simulink model "Chem_E_Car_System_LDR_PT"  (R2026a)
settings: Solver=VariableStepAuto  AbsTol=1e-3
libraries: fl_lib x32, ElectroChem_lib x10, nesl_utility x9, ee_lib x7, batteryecm_lib x1, batt_lib x1, sdl_lib x1
settings Model: Creator=eyede  LastModifiedBy=davin
settings DebuggingCC: SymbolicDimsDataTypeCodeGenerationDiagnostic=none
settings SimscapeCC: SimscapeNominalValues="[{\"value\":\"1\",\"unit\":\"A\"},{\"value\":\"1\",\"unit\":\"bar\"},{\"value\":\"1\",\"unit\":\"cm^2\"},{\"value\":\"1\",\"unit\":\"cm^3/s\"},{\"value\":\"1\",\"unit\":\"kJ/kg\"},{\"value\":\"1\",\"unit\":\"kW\"},{\"value\":\"1\",\"unit\":\"l\"},{\"value\":\"1\",\"unit\":\"N\"},{\"value\":\"1\",\"unit\":\"N*m\"},{\"value\":\"1\",\"unit\":\"V\"}]"  SimscapeLogSimulationStatistics=on

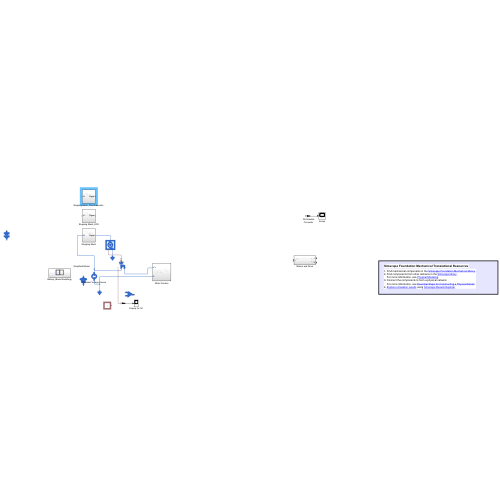
[thumbnail: Simulink's stored preview of the top-level diagram]
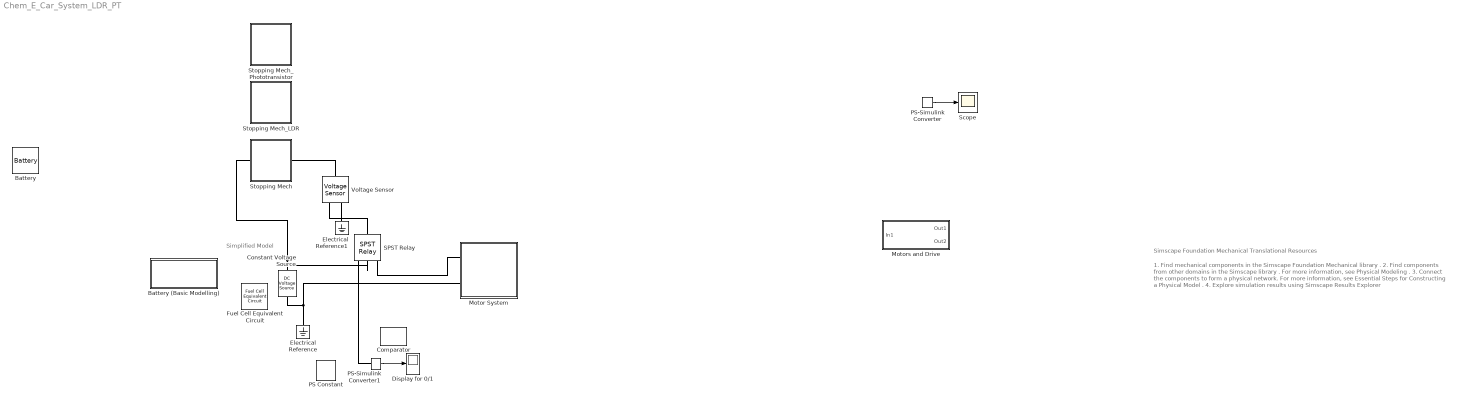
== system Chem_E_Car_System_LDR_PT ==
  note: Simplified Model
  note: 1. Find mechanical components in the Simscape Foundation Mechanical library .
      | 2. Find components from other domains in the Simscape library .
      | For more information, see Physical Modeling .
      | 3. Connect the components to form a physical network.
      | For more information, see Essential Steps for Constructing a Physical Model .
      | 4. Explore simulation results using Simscape Results Explorer
  note: Simscape Foundation Mechanical Translational Resources
  Battery : batteryecm_lib/Battery  Vnom=12 V  prm_dir=simscape.enum.battery.prm_dir.disabled  R1_dis=2 Ohm  R1_ch=2 Ohm  R1=2 Ohm  prm_AH=simscape.enum.battery.prm_AH.infinite  AH=50 A*hr  V1=11.5 V  AH1=25 A*hr  prm_R2=simscape.enum.battery.prm_R2.disabled  R2=2000 Ohm  Tmeas=298.15 K  charge_measurement_port=simscape.enum.battery.enable.no  prm_dyn=simscape.enum.battery.prm_dyn.off  Rp1=0.005 Ohm  tau1=30 s  Rp2=0.005 Ohm  tau2=30 s  Rp3=0.005 Ohm  tau3=30 s  Rp4=0.005 Ohm  tau4=30 s  Rp5=0.005 Ohm  tau5=30 s  prm_fade=simscape.enum.battery.prm_fade.disabled  N_fade=100  AH_fade=45 A*hr  R1_fade=2.02 Ohm  R1_ch_fade=2.02 Ohm  V1_fade=10.35 V  prm_age=simscape.enum.battery.prm_age.disabled  prm_age_OCV=simscape.enum.battery.prm_age_OCV.OCV  OCV_age=0.9  SOC_age=60  Tmeas_age=298.15 K  delta_time_age_vec=[0] d  temperature_age_vec=[273] K  OCV_scaling_age=2.2134e6  OCV_offset_age=1.632e6  temp_exp_age=0.515833569 V  t_exp_age=0.75  Vnom_T2=12 V  R1_T2=2.2 Ohm  R1_T2_dis=2.2 Ohm  R1_T2_ch=2.2 Ohm  V1_T2=11.4 V  R2_T2=2200 Ohm  Rp1_T2=0.005 Ohm  tau1_T2=30 s  Rp2_T2=0.005 Ohm  tau2_T2=30 s  Rp3_T2=0.005 Ohm  tau3_T2=30 s  Rp4_T2=0.005 Ohm  tau4_T2=30 s  Rp5_T2=0.005 Ohm  tau5_T2=30 s  Tmeas2=273.15 K  thermal_port=simscape.enum.thermaleffects.omit  thermal_mass=30000 J/K  i_specify=off  i_priority=None  i=0 A  i_nominal_specify=off  i_nominal_value=1  i_nominal_unit=A  v_specify=off  v_priority=None  v=0 V  v_nominal_specify=off  v_nominal_value=1  v_nominal_unit=V  charge_specify=off  charge_priority=High  charge=50 A*hr  charge_nominal_specify=off  charge_nominal_value=1  charge_nominal_unit=A*hr  num_cycles_specify=off  num_cycles_priority=High  num_cycles=0  num_cycles_nominal_specify=off  num_cycles_nominal_value=1  num_cycles_nominal_unit=1  temperature_specify=off  temperature_priority=High  temperature=298.15 K  temperature_nominal_specify=off  temperature_nominal_value=1  temperature_nominal_unit=K
  Battery (Basic Modelling) : Subsystem
  Comparator : ee_lib/Integrated Circuits/Comparator  V_OS=5 mV  C_IN=0 pF  V_OL=0 V  V_OH=5 V  R_OUT=50 Ohm  Delay=0 s
  Constant Voltage Source : ee_lib/Additional Components/SPICE Sources/DC Voltage Source  DC=6 V
  Display for 0/1 : Display
  Electrical Reference : fl_lib/Electrical/Electrical Elements/Electrical Reference
  Electrical Reference1 : fl_lib/Electrical/Electrical Elements/Electrical Reference
  Fuel Cell Equivalent Circuit : batt_lib/Cells/Fuel Cell Equivalent Circuit  Area=14.8 cm^2  NominalPotential=6 V  VoltageRange=[0, inf] V  TafelSlope=0.0136 V  NominalExchangeCurrent=0.04777 A  EquivalentResistanceRC=5e-3 Ohm  TimeConstantRC=100 s  Thickness=0.127 mm  Density=1.9 g/cm^3  MolarMass=1400 g/mol  NumSlices=3  MoistureSpec=simscape.battery.enum.cells.MoistureSpec.lambda  LambdaInterface=simscape.battery.enum.cells.BlockInterface.parameters  RHAnodeParameter=1  RHCathodeParameter=1  LambdaAnodeParameter=1  LambdaCathodeParameter=1  InitialRH=1  InitialLambda=1  DiffusionInterface=simscape.battery.enum.cells.BlockCoefficientInterface.parameters  DiffusionCoefficient=1.5e-10 m^2/s  DiffusionTableData=[1e-10, 1.5e-10] m^2/s  DiffusionBreakpoints=[0, 400] K  DragInterface=simscape.battery.enum.cells.BlockCoefficientInterface.parameters  DragCoefficient=2.5  DragTableData=[1, 2.5, 2.5]  DragBreakpoints=[1, 14, 20]  DragScaleFactor=1  TemperatureInterface=simscape.battery.enum.cells.BlockInterface.parameters  CellTemperatureParameter=303.15 K  fuelCellVoltage_specify=off  fuelCellVoltage_priority=None  fuelCellVoltage=0 V  fuelCellVoltage_nominal_specify=off  fuelCellVoltage_nominal_value=1  fuelCellVoltage_nominal_unit=V  fuelCellCurrent_specify=off  fuelCellCurrent_priority=None  fuelCellCurrent=0 A  fuelCellCurrent_nominal_specify=off  fuelCellCurrent_nominal_value=1  fuelCellCurrent_nominal_unit=A
  Motor System : Subsystem
  Motors and Drive : Subsystem
  PS Constant : fl_lib/Physical Signals/Sources/PS Constant  constant=1
  PS-Simulink Converter : nesl_utility/PS-Simulink Converter  PhysicalDomain=network_engine_domain  SubClassName=ps_output  LeftPortType=input  RightPortType=output  PseudoPeriodic=off  Frequencies=[]  VectorFormat=inherit  Unit=inherit  AffineConversion=off
  PS-Simulink Converter1 : nesl_utility/PS-Simulink Converter  PhysicalDomain=network_engine_domain  SubClassName=ps_output  LeftPortType=input  RightPortType=output  PseudoPeriodic=off  Frequencies=[]  VectorFormat=inherit  Unit=inherit  AffineConversion=off
  SPST Relay : ee_lib/Switches & Breakers/Relays/SPST Relay  block_choices=ee.enum.controlport.ps  R_closed=0 Ohm  G_open=1e-8 1/Ohm  Threshold=1  exposemeasurement=ee.enum.exposemeasurement.visible  V_rated=5 V  V_energize=75  V_deenergize=25  l_winding=0.08 H  r_winding=12.5 Ohm  g_winding=1e-9 1/Ohm  T_brk_C_S=0 s  T_mak_C_S=0 s  fault_types=ee.enum.relays.faultTypes.winding
  Scope : Scope
  Stopping Mech : Subsystem
  Stopping Mech_LDR : Subsystem
  "Stopping Mech_Phototransistor " : Subsystem
  Voltage Sensor : fl_lib/Electrical/Electrical Sensors/Voltage Sensor
  wires:
  PS-Simulink Converter/1 -> Scope/1
  PS-Simulink Converter1/1 -> Display for 0/1/1
  connections:
  Electrical Reference/LConn1 -- Motor System/LConn2 -- Constant Voltage Source/RConn1
  Voltage Sensor/LConn1 -- Stopping Mech/RConn1
  SPST Relay/RConn1 -- Motor System/LConn1
  SPST Relay/RConn2 -- Stopping Mech/LConn1 -- Constant Voltage Source/LConn1
  Voltage Sensor/RConn1 -- SPST Relay/LConn1
  Electrical Reference1/LConn1 -- Voltage Sensor/RConn2
  PS-Simulink Converter1/LConn1 -- SPST Relay/RConn3

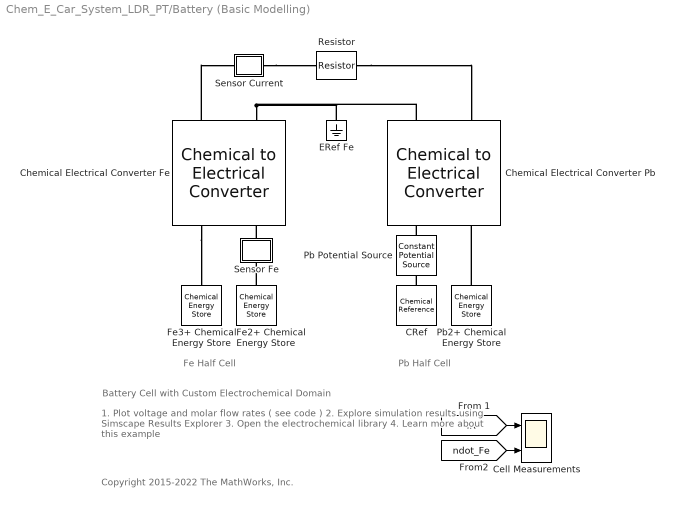
== system Chem_E_Car_System_LDR_PT/Battery (Basic Modelling) ==
  note: 1. Plot voltage and molar flow rates ( see code )
      | 2. Explore simulation results using Simscape Results Explorer
      | 3. Open the electrochemical library
      | 4. Learn more about this example
  note: Battery Cell with Custom Electrochemical Domain
  note: Copyright 2015-2022 The MathWorks, Inc.
  note: Pb Half Cell
  note: Fe Half Cell
  CRef : ElectroChem_lib/Electrochemical Elements/Chemical Reference
  Cell Measurements : Scope  NumInputPorts=2
      settings: Title=Battery Current (A)  ActiveDisplayYMinimum=-0.0017010196663266859  ActiveDisplayYMaximum=100  DataLoggingSaveFormat=Array
  Chemical Electrical Converter Fe : ElectroChem_lib/Electrochemical Elements/Chemical to Electrical Converter  z=1  i_specify=off  i_priority=High  i=0 A  i_nominal_specify=off  i_nominal_value=1  i_nominal_unit=A  ndot_specify=off  ndot_priority=High  ndot=0 mol/s  ndot_nominal_specify=off  ndot_nominal_value=1  ndot_nominal_unit=mol/s
  Chemical Electrical Converter Pb : ElectroChem_lib/Electrochemical Elements/Chemical to Electrical Converter  z=2  i_specify=off  i_priority=High  i=0 A  i_nominal_specify=off  i_nominal_value=1  i_nominal_unit=A  ndot_specify=off  ndot_priority=High  ndot=0 mol/s  ndot_nominal_specify=off  ndot_nominal_value=1  ndot_nominal_unit=mol/s
  ERef Fe : fl_lib/Electrical/Electrical Elements/Electrical Reference
  Fe2+ Chemical Energy Store : ElectroChem_lib/Electrochemical Elements/Chemical Energy Store  mu0=-78.87e3 J/mol  m_solvent=1 kg  T=298 K  ndot_specify=off  ndot_priority=High  ndot=0 mol/s  ndot_nominal_specify=off  ndot_nominal_value=1  ndot_nominal_unit=mol/s  n_specify=on  n_priority=High  n=0.01 mol  n_nominal_specify=off  n_nominal_value=1  n_nominal_unit=mol
  Fe3+ Chemical Energy Store : ElectroChem_lib/Electrochemical Elements/Chemical Energy Store  mu0=-4.60e3 J/mol  m_solvent=1 kg  T=298 K  ndot_specify=off  ndot_priority=High  ndot=0 mol/s  ndot_nominal_specify=off  ndot_nominal_value=1  ndot_nominal_unit=mol/s  n_specify=on  n_priority=High  n=0.05 mol  n_nominal_specify=off  n_nominal_value=1  n_nominal_unit=mol
  Pb Potential Source : ElectroChem_lib/Electrochemical Sources/Constant Potential Source  mu0=0 J/mol
  Pb2+ Chemical Energy Store : ElectroChem_lib/Electrochemical Elements/Chemical Energy Store  mu0=-24.39e3 J/mol  m_solvent=1 kg  T=298 K  ndot_specify=off  ndot_priority=High  ndot=0 mol/s  ndot_nominal_specify=off  ndot_nominal_value=1  ndot_nominal_unit=mol/s  n_specify=on  n_priority=High  n=0.1 mol  n_nominal_specify=off  n_nominal_value=1  n_nominal_unit=mol
  Resistor : fl_lib/Electrical/Electrical Elements/Resistor  R=0.012 Ohm  i_specify=off  i_priority=High  i=0 A  i_nominal_specify=off  i_nominal_value=1  i_nominal_unit=A  v_specify=off  v_priority=High  v=0 V  v_nominal_specify=off  v_nominal_value=1  v_nominal_unit=V
  Sensor Current : Subsystem
      mask Display: disp('iR')
  Sensor Fe : Subsystem
      mask Display: disp('ndot')
  wires:
  [ndot_Fe] -> Cell Measurements/2
  [iR] -> Cell Measurements/1
  connections:
  Chemical Electrical Converter Fe/LConn2 -- ERef Fe/LConn1 -- Chemical Electrical Converter Pb/LConn2
  Pb Potential Source/LConn1 -- Chemical Electrical Converter Pb/RConn2
  Resistor/RConn1 -- Chemical Electrical Converter Pb/LConn1
  Chemical Electrical Converter Fe/RConn1 -- Fe3+ Chemical Energy Store/LConn1
  CRef/LConn1 -- Pb Potential Source/RConn1
  Fe2+ Chemical Energy Store/LConn1 -- Sensor Fe/RConn1
  Chemical Electrical Converter Fe/LConn1 -- Sensor Current/LConn1
  Sensor Fe/LConn1 -- Chemical Electrical Converter Fe/RConn2
  Sensor Current/RConn1 -- Resistor/LConn1
  Pb2+ Chemical Energy Store/LConn1 -- Chemical Electrical Converter Pb/RConn1

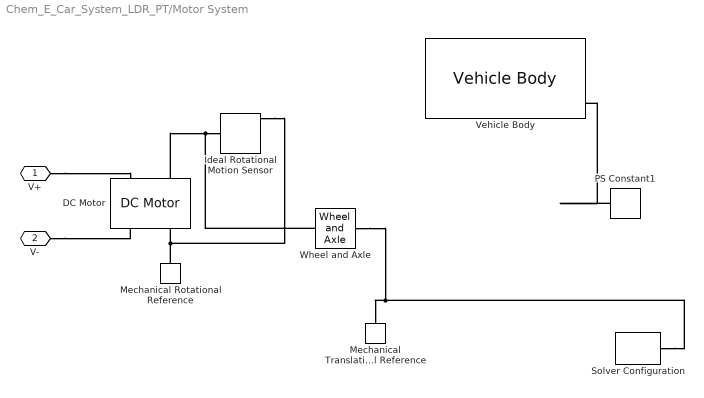
== system Chem_E_Car_System_LDR_PT/Motor System ==
  DC Motor : ee_lib/Electromechanical/Brushed Motors/DC Motor  field_option=ee.enum.field_option.pm  Rf=100 Ohm  Lf=1 H  Laf=0.15 H  If0=0 A  parameterization=ee.enum.dcparam_option.circuit_param  Ra=3.9 Ohm  La=12e-6 H  emf_or_torque=ee.enum.emf_or_torque.kv  Kv=0.072e-3 V/rpm  Ki=6.876e-4 N*m/A  T_stall=0.24e-3 N*m  w_max=19100 rpm  w_rated=15000 rpm  P_rated=0.08 W  V_rated=1.5 V  lam_param=ee.enum.lam_param.damping  i_noload=0 A  V_i_noload=1.5 V  J=0.01 cm^2*g  lam=0 N*m*s/rad  speed0=0 rpm  alpha=3.93e-3 1/K  Tmeas=25 degC  thermal_mass=100 J/K  initial_temperature=25 degC
  Ideal Rotational Motion Sensor : fl_lib/Mechanical/Mechanical Sensors/Ideal Rotational Motion Sensor  reference=foundation.enum.MeasurementReference.difference  acceleration_port=false  velocity_port=true  position_port=true  wrap_angle=false  offset=0 rad
  Mechanical Rotational Reference : fl_lib/Mechanical/Rotational Elements/Mechanical Rotational Reference
  Mechanical Translational Reference : fl_lib/Mechanical/Translational Elements/Mechanical Translational Reference
  PS Constant1 : fl_lib/Physical Signals/Sources/PS Constant  constant=0
  Solver Configuration : nesl_utility/Solver Configuration  PhysicalDomain=network_engine_domain  SubClassName=solver  LeftPortType=input  RightPortType=generic  Tones=[]  Harmonics=[]  SimulateNoise=off  Profile=off  UseLocalSampling=off  EnableSwitchedLinearOptims=on  FrequencyDomain=off  UseCCode=off  RelTol=0.001  AbsTol=1e-06  MinStep=1e-09  ToWorkspace=off  RevertToSquareIcSolve=off  NumHomotopyIterations=100  PhasorMode=off  PhasorModeNumHarmonics=1  ConsistencySolver=NEWTON_XTOL_AFTER_FTOL  CanonicalOrdering=UNORDERED  OptimizeIntermediates=UNOPTIMIZED  IndexReductionMethod=DerivativeReplacement  DoDC=off  ResidualTolerance=1e-09  ConsistencyTolSource=GLOBAL  ConsistencyAbsTol=0.001  ConsistencyRelTol=0.001  ConsistencyTolFactor=0.001  UseLocalSolver=off  LocalSolverChoice=NE_BACKWARD_EULER_ADVANCER  ResolveIndetEquations=on  FunctionEvalNumThread=1  LocalSolverSampleTime=0.001  DoFixedCost=off  MaxNonlinIter=3  MaxModeIter=2  ComputeImpulses=off  ImpulseIterations=2  LinearAlgebra=auto  LinearAlgebraNumThread=0  EquationFormulation=NE_TIME_EF  DelaysMemoryBudget=1024  AutomaticFiltering=on  FilteringTimeConstant=0.001  PartitionStorageMethod=AS_NEEDED  PartitionMemoryBudget=1024  PartitionMethod=ROBUST  MultibodyUseLocalSolver=off  MultibodyLocalSolverChoice=ODE1  MultibodyLocalSolverSampleTime=0.001
  Vehicle Body : sdl_lib/Tires & Vehicles/Vehicle Body  mass=1200 kg  n_w=2  x_f=1.4 m  x_r=1.6 m  y_c=0.5 m  mass_var=false  g=9.81 m/s^2  liftoff_warning=false  area=3 m^2  Cd_var=false  Cd=0.4  rho=1.18 kg/m^3  model_pitch=false  inertia=4000 kg*m^2  suspension_model=sdl.enum.linearTLU.linear  k_f=1e4 N/m  b_f=1e4 N*s/m  k_r=1e4 N/m  b_r=1e4 N*s/m  k_f_TLU=[-2000, -1000, 0, 1000, 2000] N  x_f_TLU=[-.4, -.2, 0, .2, .4] m  b_f_TLU=[-200, -100, 0, 100, 200] N  v_f_TLU=[-4, -2, 0, 2, 4] m/s  k_r_TLU=[-2000, -1000, 0, 1000, 2000] N  x_r_TLU=[-.4, -.2, 0, .2, .4] m  b_r_TLU=[-200, -100, 0, 100, 200] N  v_r_TLU=[-4, -2, 0, 2, 4] m/s  interp_method=simscape.enum.interpolation.linear  extrap_method=simscape.enum.extrapolation.linear  model_hardstop=false  upper_bound_f=.25 m  lower_bound_f=-.25 m  stop_k_f=1e6 N/m  stop_b_f=150 N*s/m  upper_bound_r=.25 m  lower_bound_r=-.25 m  stop_k_r=1e6 N/m  stop_b_r=150 N*s/m  initial_pitch=0 rad  initial_pitch_rate=0 rad/s  v_specify=off  v_priority=High  v=0 m/s  v_nominal_specify=off  v_nominal_value=1  v_nominal_unit=m/s
  Wheel and Axle : fl_lib/Mechanical/Mechanisms/Wheel and Axle  R=0.05 m  or=foundation.enum.DriveOrientation.Positive  t_specify=off  t_priority=None  t=0 N*m  t_nominal_specify=off  t_nominal_value=1  t_nominal_unit=N*m  f_specify=off  f_priority=None  f=0 N  f_nominal_specify=off  f_nominal_value=1  f_nominal_unit=N
  V+ : PMIOPort  Side=Left
  V- : PMIOPort  Port=2  Side=Left
  connections:
  DC Motor/RConn2 -- Mechanical Rotational Reference/LConn1 -- Ideal Rotational Motion Sensor/RConn1
  Ideal Rotational Motion Sensor/LConn1 -- DC Motor/LConn2 -- Wheel and Axle/LConn1
  Solver Configuration/RConn1 -- Wheel and Axle/RConn1 -- Mechanical Translational Reference/LConn1
  PS Constant1/RConn1 -- Vehicle Body/RConn3
  V+/RConn1 -- DC Motor/LConn1
  V-/RConn1 -- DC Motor/RConn1

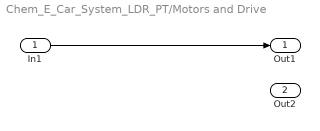
== system Chem_E_Car_System_LDR_PT/Motors and Drive ==
  In1 : Inport
  Out1 : Outport
  Out2 : Outport  Port=2
  wires:
  In1/1 -> Out1/1

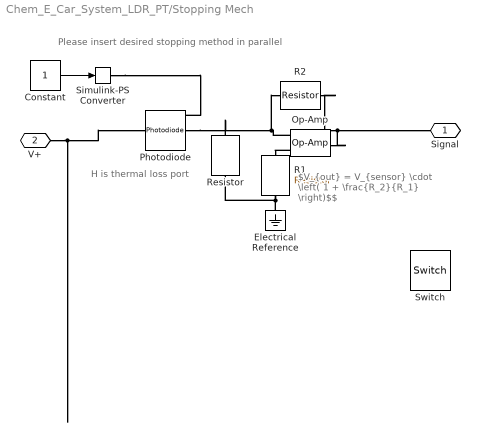
== system Chem_E_Car_System_LDR_PT/Stopping Mech ==
  note: $V_{out} = V_{sensor} \cdot \left( 1 + \frac{R_2}{R_1} \right)$$
  note: H is thermal loss port
  note: Please insert desired stopping method in parallel
  Constant : Constant
  Electrical Reference : fl_lib/Electrical/Electrical Elements/Electrical Reference
  Op-Amp : fl_lib/Electrical/Electrical Elements/Op-Amp  outI_specify=off  outI_priority=None  outI=0 A  outI_nominal_specify=off  outI_nominal_value=1  outI_nominal_unit=A
  Photodiode : ee_lib/Sensors & Transducers/Photodiode  prmFlux=ee.enum.diode.photodiodeFlux.fluxDensity  Imeas=25 uA  FluxD=5 W/m^2  G=5e-6 A*m^2/W  prmExp=ee.enum.diode.photodiode.useIVIs  I2=0.1 A  V2=1.3 V  IS=5e-9 A  ec=3  RS=0.1 Ohm  Tmeas=25 degC  C_param=ee.enum.diode.capParam.fixed  CJ=60 pF  CJ0=60 pF  Vvec=[.1, 10, 100] V  Cvec=[45, 3, 6] pF  VJ=1 V  Mgrad=0.5  FC=0.5  T_param=ee.enum.diode.temperatureParam.off  Tdevice=25 degC  IS_T2=2.5e-7 A  I1_T2=0.07 A  V1_T2=1.3 V  Tmeas2=125 degC  EG_param=ee.enum.diode.egapParam.material_si  EG=1.11 eV  XTI_param=ee.enum.diode.xtiParam.pn  XTI=3  i_specify=off  i_priority=None  i=0 A  i_nominal_specify=off  i_nominal_value=1  i_nominal_unit=A  v_specify=off  v_priority=None  v=0 V  v_nominal_specify=off  v_nominal_value=1  v_nominal_unit=V  v_capacitor_specify=off  v_capacitor_priority=None  v_capacitor=0 V  v_capacitor_nominal_specify=off  v_capacitor_nominal_value=1  v_capacitor_nominal_unit=V  Qj_specify=off  Qj_priority=High  Qj=0 C  Qj_nominal_specify=off  Qj_nominal_value=1  Qj_nominal_unit=C  thermal_network_parameterization=ee.enum.thermalNetworkTopology.junctionCase  Rth=[0, 10] K/W  Rth_Cauer=[1, 3, 10] K/W  Rth_Foster=[.08, .14, .22, .16] K/W  thermal_mass_parameterization=ee.enum.thermalNetwork.timeconstant  thermal_mass=[0, 1] J/K  thermal_mass_Cauer=[1.5, 2, 3] J/K  thermal_mass_Foster=[.001, .005, .05, .5] J/K  thermal_time_constant=[0, 10] s  thermal_time_constant_Cauer=[1, 3, 10] s  thermal_time_constant_Foster=[7e-05, .0007, .01, .08] s  thermal_mass_initial_temperatures=[25, 25] degC  thermal_mass_initial_temperatures_Cauer=[25, 25, 25] degC  steadyState_Foster=simscape.enum.onoff.on  Tvec_initial_Foster=[25, 25, 25, 25] degC
  R1 : fl_lib/Electrical/Electrical Elements/Resistor  R=10 kOhm  i_specify=off  i_priority=None  i=0 A  i_nominal_specify=off  i_nominal_value=1  i_nominal_unit=A  v_specify=off  v_priority=None  v=0 V  v_nominal_specify=off  v_nominal_value=1  v_nominal_unit=V
  R2 : fl_lib/Electrical/Electrical Elements/Resistor  R=90 kOhm  i_specify=off  i_priority=None  i=0 A  i_nominal_specify=off  i_nominal_value=1  i_nominal_unit=A  v_specify=off  v_priority=None  v=0 V  v_nominal_specify=off  v_nominal_value=1  v_nominal_unit=V
  Resistor : fl_lib/Electrical/Electrical Elements/Resistor  R=100 kOhm  i_specify=off  i_priority=None  i=0 A  i_nominal_specify=off  i_nominal_value=1  i_nominal_unit=A  v_specify=off  v_priority=None  v=0 V  v_nominal_specify=off  v_nominal_value=1  v_nominal_unit=V
  Simulink-PS Converter : nesl_utility/Simulink-PS Converter  PhysicalDomain=network_engine_domain  SubClassName=ps_input  LeftPortType=input  RightPortType=output  PseudoPeriodic=off  Frequencies=[]  NoiseDistribution=none  NoiseParameters=[]  Unit=1  AffineConversion=off  FilteringAndDerivatives=provide  SimscapeFilterOrder=1  InputFilterTimeConstant=0.001  UdotUserProvided=0
  Switch : fl_lib/Electrical/Electrical Elements/Switch  R_closed=0.01 Ohm  G_open=1e-8 1/Ohm  Threshold=0.5  i_specify=off  i_priority=None  i=0 A  i_nominal_specify=off  i_nominal_value=1  i_nominal_unit=A  v_specify=off  v_priority=None  v=0 V  v_nominal_specify=off  v_nominal_value=1  v_nominal_unit=V
  Signal : PMIOPort  Side=Right
  V+ : PMIOPort  Port=2  Side=Left
  wires:
  Constant/1 -> Simulink-PS Converter/1
  connections:
  Simulink-PS Converter/RConn1 -- Photodiode/LConn1
  V+/RConn1 -- Photodiode/RConn1
  R2/RConn1 -- Op-Amp/RConn1 -- Signal/RConn1
  Electrical Reference/LConn1 -- Resistor/RConn1 -- R1/RConn1
  Op-Amp/LConn1 -- R1/LConn1
  Op-Amp/LConn2 -- Resistor/LConn1 -- Photodiode/LConn2 -- R2/LConn1

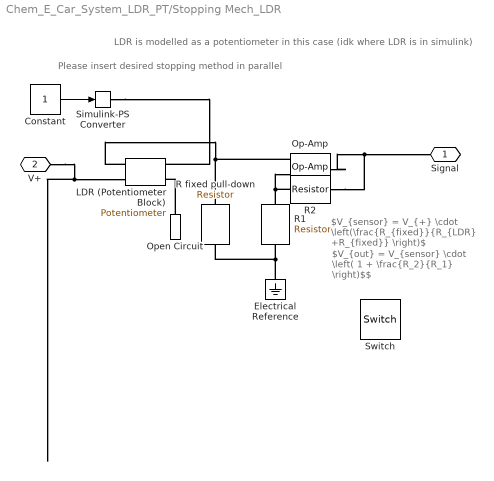
== system Chem_E_Car_System_LDR_PT/Stopping Mech_LDR ==
  note: $V_{sensor} = V_{+} \cdot \left(\frac{R_{fixed}}{R_{LDR} +R_{fixed}} \right)$
  note: Please insert desired stopping method in parallel
  note: LDR is modelled as a potentiometer in this case (idk where LDR is in simulink)
  note: $V_{out} = V_{sensor} \cdot \left( 1 + \frac{R_2}{R_1} \right)$$
  Constant : Constant
  Electrical Reference : fl_lib/Electrical/Electrical Elements/Electrical Reference
  LDR (Potentiometer Block) : ee_lib/Passive/Potentiometer  nPorts=ee.enum.passive.potentiometer.nPorts.Three  R0=1000 Ohm  Rw=1 Ohm  xmin=0  xmax=1  minResistance=1 Ohm  maxResistance=999 Ohm  xmin2port=0  xmax2port=1  Taper=ee.enum.passive.potentiometer.linOrLog.lin  Rcenter=200 Ohm  Gradient=ee.enum.passive.potentiometer.gradient.higherR
  Op-Amp : fl_lib/Electrical/Electrical Elements/Op-Amp  outI_specify=off  outI_priority=None  outI=0 A  outI_nominal_specify=off  outI_nominal_value=1  outI_nominal_unit=A
  Open Circuit : fl_lib/Electrical/Electrical Elements/Open Circuit  v_specify=off  v_priority=None  v=0 V  v_nominal_specify=off  v_nominal_value=1  v_nominal_unit=V
      settings: LibrarySourceBlock=|
      | ee_lib/Connectors &
      | References/Open Circuit
  R fixed pull-down : fl_lib/Electrical/Electrical Elements/Resistor  R=100 kOhm  i_specify=off  i_priority=None  i=0 A  i_nominal_specify=off  i_nominal_value=1  i_nominal_unit=A  v_specify=off  v_priority=None  v=0 V  v_nominal_specify=off  v_nominal_value=1  v_nominal_unit=V
  R1 : fl_lib/Electrical/Electrical Elements/Resistor  R=10 kOhm  i_specify=off  i_priority=None  i=0 A  i_nominal_specify=off  i_nominal_value=1  i_nominal_unit=A  v_specify=off  v_priority=None  v=0 V  v_nominal_specify=off  v_nominal_value=1  v_nominal_unit=V
  R2 : fl_lib/Electrical/Electrical Elements/Resistor  R=90 kOhm  i_specify=off  i_priority=None  i=0 A  i_nominal_specify=off  i_nominal_value=1  i_nominal_unit=A  v_specify=off  v_priority=None  v=0 V  v_nominal_specify=off  v_nominal_value=1  v_nominal_unit=V
  Simulink-PS Converter : nesl_utility/Simulink-PS Converter  PhysicalDomain=network_engine_domain  SubClassName=ps_input  LeftPortType=input  RightPortType=output  PseudoPeriodic=off  Frequencies=[]  NoiseDistribution=none  NoiseParameters=[]  Unit=1  AffineConversion=off  FilteringAndDerivatives=provide  SimscapeFilterOrder=1  InputFilterTimeConstant=0.001  UdotUserProvided=0
  Switch : fl_lib/Electrical/Electrical Elements/Switch  R_closed=0.01 Ohm  G_open=1e-8 1/Ohm  Threshold=0.5  i_specify=off  i_priority=None  i=0 A  i_nominal_specify=off  i_nominal_value=1  i_nominal_unit=A  v_specify=off  v_priority=None  v=0 V  v_nominal_specify=off  v_nominal_value=1  v_nominal_unit=V
  Signal : PMIOPort  Side=Right
  V+ : PMIOPort  Port=2  Side=Left
  wires:
  Constant/1 -> Simulink-PS Converter/1
  connections:
  Simulink-PS Converter/RConn1 -- LDR (Potentiometer Block)/RConn2
  V+/RConn1 -- LDR (Potentiometer Block)/LConn1
  R2/RConn1 -- Op-Amp/RConn1 -- Signal/RConn1
  Electrical Reference/LConn1 -- R1/RConn1 -- R fixed pull-down/RConn1
  LDR (Potentiometer Block)/LConn2 -- Op-Amp/LConn1 -- R fixed pull-down/LConn1
  R1/LConn1 -- R2/LConn1 -- Op-Amp/LConn2
  Open Circuit/LConn1 -- LDR (Potentiometer Block)/RConn1

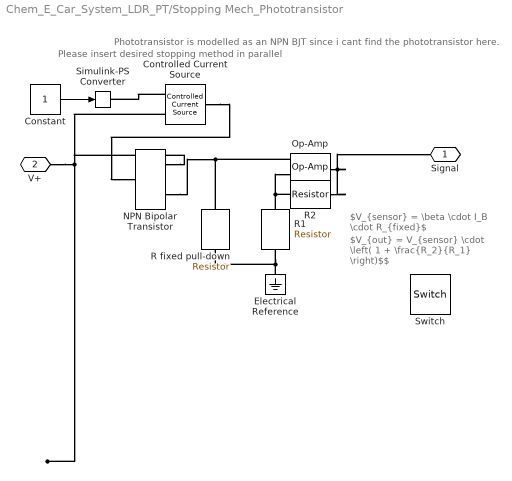
== system Chem_E_Car_System_LDR_PT/Stopping Mech_Phototransistor  ==
  note: Phototransistor is modelled as an NPN BJT since i cant find the phototransistor here.
  note: Please insert desired stopping method in parallel
  note: $V_{sensor} = \beta \cdot I_B \cdot R_{fixed}$
  note: $V_{out} = V_{sensor} \cdot \left( 1 + \frac{R_2}{R_1} \right)$$
  Constant : Constant
  Controlled Current Source : fl_lib/Electrical/Electrical Sources/Controlled Current Source
  Electrical Reference : fl_lib/Electrical/Electrical Elements/Electrical Reference
  NPN Bipolar Transistor : ee_lib/Semiconductors & Converters/NPN Bipolar Transistor  parameterization=1  BF=100  IS=1e-14 A  VAF=200 V  hfe=100  hoe=50e-6 1/Ohm  Ic_h=1 mA  Vce_h=5 V  V1=0.55 V  I1=0.5 mA  BR=1  Tmeas=25 degC  RC=0.01 Ohm  RE=1e-4 Ohm  RB=1 Ohm  C_BC=5 pF  C_BE=5 pF  TF=0 us  TR=0 us  prmDatasheet=1  prmEquCoeff=1  hfe_T2=125  XTB=0  V1_T2=0.45 V  I1_T2=0.5 mA  Tmeas2=125 degC  EG=1.11 eV  XTI=3  TdeviceDatasheet=25 degC  TdeviceEquCoeff=25 degC  ec=1  ib_specify=off  ib_priority=None  ib=0 A  ib_nominal_specify=off  ib_nominal_value=1  ib_nominal_unit=A  ic_specify=off  ic_priority=None  ic=0 A  ic_nominal_specify=off  ic_nominal_value=1  ic_nominal_unit=A  vce_specify=off  vce_priority=None  vce=0 V  vce_nominal_specify=off  vce_nominal_value=1  vce_nominal_unit=V  vbe_specify=off  vbe_priority=None  vbe=0 V  vbe_nominal_specify=off  vbe_nominal_value=1  vbe_nominal_unit=V  Qbc_specify=off  Qbc_priority=High  Qbc=0 C  Qbc_nominal_specify=off  Qbc_nominal_value=1  Qbc_nominal_unit=uC  Qbe_specify=off  Qbe_priority=High  Qbe=0 C  Qbe_nominal_specify=off  Qbe_nominal_value=1  Qbe_nominal_unit=uC  thermal_network_parameterization=ee.enum.thermalNetworkTopology.junctionCase  Rth=[0, 10] K/W  Rth_Cauer=[1, 3, 10] K/W  Rth_Foster=[.08, .14, .22, .16] K/W  thermal_mass_parameterization=ee.enum.thermalNetwork.timeconstant  thermal_mass=[0, 1] J/K  thermal_mass_Cauer=[.1, .3, 1] J/K  thermal_mass_Foster=[.001, .005, .05, .5] J/K  thermal_time_constant=[0, 10] s  thermal_time_constant_Cauer=[1, 3, 10] s  thermal_time_constant_Foster=[7e-05, .0007, .01, .08] s  thermal_mass_initial_temperatures=[25, 25] degC  thermal_mass_initial_temperatures_Cauer=[25, 25, 25] degC  Tvec_initial_Foster=[25, 25, 25, 25] degC
  Op-Amp : fl_lib/Electrical/Electrical Elements/Op-Amp  outI_specify=off  outI_priority=None  outI=0 A  outI_nominal_specify=off  outI_nominal_value=1  outI_nominal_unit=A
  R fixed pull-down : fl_lib/Electrical/Electrical Elements/Resistor  R=100 kOhm  i_specify=off  i_priority=None  i=0 A  i_nominal_specify=off  i_nominal_value=1  i_nominal_unit=A  v_specify=off  v_priority=None  v=0 V  v_nominal_specify=off  v_nominal_value=1  v_nominal_unit=V
  R1 : fl_lib/Electrical/Electrical Elements/Resistor  R=10 kOhm  i_specify=off  i_priority=None  i=0 A  i_nominal_specify=off  i_nominal_value=1  i_nominal_unit=A  v_specify=off  v_priority=None  v=0 V  v_nominal_specify=off  v_nominal_value=1  v_nominal_unit=V
  R2 : fl_lib/Electrical/Electrical Elements/Resistor  R=90 kOhm  i_specify=off  i_priority=None  i=0 A  i_nominal_specify=off  i_nominal_value=1  i_nominal_unit=A  v_specify=off  v_priority=None  v=0 V  v_nominal_specify=off  v_nominal_value=1  v_nominal_unit=V
  Simulink-PS Converter : nesl_utility/Simulink-PS Converter  PhysicalDomain=network_engine_domain  SubClassName=ps_input  LeftPortType=input  RightPortType=output  PseudoPeriodic=off  Frequencies=[]  NoiseDistribution=none  NoiseParameters=[]  Unit=1  AffineConversion=off  FilteringAndDerivatives=provide  SimscapeFilterOrder=1  InputFilterTimeConstant=0.001  UdotUserProvided=0
  Switch : fl_lib/Electrical/Electrical Elements/Switch  R_closed=0.01 Ohm  G_open=1e-8 1/Ohm  Threshold=0.5  i_specify=off  i_priority=None  i=0 A  i_nominal_specify=off  i_nominal_value=1  i_nominal_unit=A  v_specify=off  v_priority=None  v=0 V  v_nominal_specify=off  v_nominal_value=1  v_nominal_unit=V
  Signal : PMIOPort  Side=Right
  V+ : PMIOPort  Port=2  Side=Left
  wires:
  Constant/1 -> Simulink-PS Converter/1
  connections:
  R1/LConn1 -- Op-Amp/LConn2 -- R2/LConn1
  Op-Amp/LConn1 -- R fixed pull-down/LConn1 -- NPN Bipolar Transistor/RConn2
  Electrical Reference/LConn1 -- R fixed pull-down/RConn1 -- R1/RConn1
  Op-Amp/RConn1 -- Signal/RConn1 -- R2/RConn1
  Controlled Current Source/RConn2 -- NPN Bipolar Transistor/RConn1 -- V+/RConn1
  Controlled Current Source/RConn1 -- Simulink-PS Converter/RConn1
  Controlled Current Source/LConn1 -- NPN Bipolar Transistor/LConn1

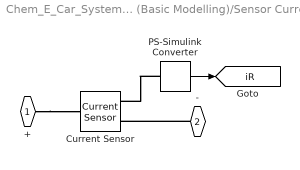
== system Chem_E_Car_System_LDR_PT/Battery (Basic Modelling)/Sensor Current ==
  Current Sensor : fl_lib/Electrical/Electrical Sensors/Current Sensor
  PS-Simulink Converter : nesl_utility/PS-Simulink Converter  PhysicalDomain=network_engine_domain  SubClassName=ps_output  LeftPortType=input  RightPortType=output  PseudoPeriodic=off  Frequencies=[]  VectorFormat=1-D array  Unit=1  AffineConversion=off
  + : PMIOPort  Side=Left
  - : PMIOPort  Port=2  Side=Right
  tag scope: iR=global
  wires:
  PS-Simulink Converter/1 -> [iR]
  connections:
  PS-Simulink Converter/LConn1 -- Current Sensor/RConn1
  +/RConn1 -- Current Sensor/LConn1
  -/RConn1 -- Current Sensor/RConn2

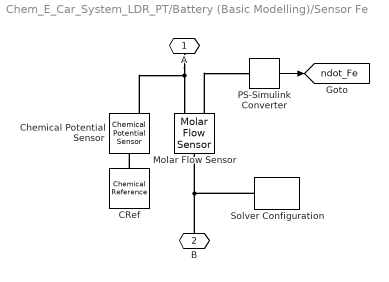
== system Chem_E_Car_System_LDR_PT/Battery (Basic Modelling)/Sensor Fe ==
  CRef : ElectroChem_lib/Electrochemical Elements/Chemical Reference
  Chemical Potential Sensor : ElectroChem_lib/Electrochemical Sensors/Chemical Potential Sensor
  Molar Flow Sensor : ElectroChem_lib/Electrochemical Sensors/Molar Flow Sensor
  PS-Simulink Converter : nesl_utility/PS-Simulink Converter  PhysicalDomain=network_engine_domain  SubClassName=ps_output  LeftPortType=input  RightPortType=output  PseudoPeriodic=off  Frequencies=[]  VectorFormat=1-D array  Unit=1  AffineConversion=off
  Solver Configuration : nesl_utility/Solver Configuration  PhysicalDomain=network_engine_domain  SubClassName=solver  LeftPortType=input  RightPortType=generic  Tones=[]  Harmonics=[]  SimulateNoise=off  Profile=off  UseLocalSampling=off  EnableSwitchedLinearOptims=on  FrequencyDomain=off  UseCCode=off  RelTol=0.001  AbsTol=1e-06  MinStep=1e-09  ToWorkspace=off  RevertToSquareIcSolve=off  NumHomotopyIterations=100  PhasorMode=off  PhasorModeNumHarmonics=1  ConsistencySolver=NEWTON_XTOL_AFTER_FTOL  CanonicalOrdering=UNORDERED  OptimizeIntermediates=UNOPTIMIZED  IndexReductionMethod=DerivativeReplacement  DoDC=off  ResidualTolerance=1e-9  ConsistencyTolSource=GLOBAL  ConsistencyAbsTol=0.001  ConsistencyRelTol=0.001  ConsistencyTolFactor=0.001  UseLocalSolver=off  LocalSolverChoice=NE_BACKWARD_EULER_ADVANCER  ResolveIndetEquations=on  FunctionEvalNumThread=1  LocalSolverSampleTime=0.001  DoFixedCost=off  MaxNonlinIter=3  MaxModeIter=2  ComputeImpulses=off  ImpulseIterations=2  LinearAlgebra=auto  LinearAlgebraNumThread=0  EquationFormulation=NE_TIME_EF  DelaysMemoryBudget=1024  AutomaticFiltering=on  FilteringTimeConstant=0.001  PartitionStorageMethod=AS_NEEDED  PartitionMemoryBudget=1024  PartitionMethod=FAST  MultibodyUseLocalSolver=off  MultibodyLocalSolverChoice=ODE1  MultibodyLocalSolverSampleTime=0.001
  A : PMIOPort  Side=Left
  B : PMIOPort  Port=2  Side=Right
  tag scope: ndot_Fe=global
  wires:
  PS-Simulink Converter/1 -> [ndot_Fe]
  connections:
  B/RConn1 -- Solver Configuration/RConn1 -- Molar Flow Sensor/RConn1
  A/RConn1 -- Chemical Potential Sensor/LConn1 -- Molar Flow Sensor/LConn1
  Molar Flow Sensor/LConn2 -- PS-Simulink Converter/LConn1
  CRef/LConn1 -- Chemical Potential Sensor/RConn1
